simulink model "RedCrane_kinematic_model_telescope"  (R2024a)
settings: Solver=FixedStepAuto  StartTime=0.0  StopTime=40  FixedStep=Ts  MaxStep=0.005  RelTol=1e-3
values from neighbouring files (symbols this model uses):
  Cartesian_home = [3.55, 0.4, 1.6]'    [enviroment_setup.m]
  telescope0 = 0    [enviroment_setup.m]
  thetaList0 = [0, 0,-pi/8, 0, 0]'    [enviroment_setup.m]
  Ts = 0.001    [enviroment_setup.m]
undefined symbols (not defined in the file or in its folder): dp_k_angle_to_stroke, dp_m_angle_to_stroke, p_k_angle_to_stroke, p_k_stroke_to_angle, p_m_angle_to_stroke, p_m_stroke_to_angle, X, Y, Z
libraries: sm_lib x82, nesl_utility x19, fl_lib x16
(part 3 of 3)

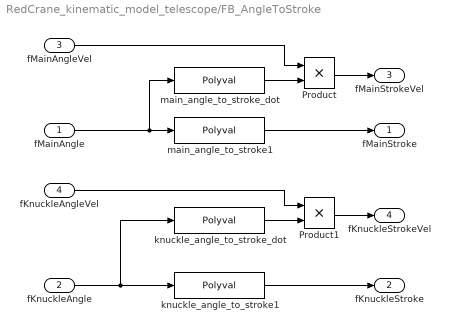
== system RedCrane_kinematic_model_telescope/FB_AngleToStroke ==
  fMainAngle : Inport
  fKnuckleAngle : Inport  Port=2
  fMainAngleVel : Inport  Port=3
  fKnuckleAngleVel : Inport  Port=4
  Product : Product
  Product1 : Product
  knuckle_angle_to_stroke1 : Polyval  Coefs=p_k_angle_to_stroke
  knuckle_angle_to_stroke_dot : Polyval  Coefs=dp_k_angle_to_stroke
  main_angle_to_stroke1 : Polyval  Coefs=p_m_angle_to_stroke
  main_angle_to_stroke_dot : Polyval  Coefs=dp_m_angle_to_stroke
  fMainStroke : Outport
  fKnuckleStroke : Outport  Port=2
  fMainStrokeVel : Outport  Port=3
  fKnuckleStrokeVel : Outport  Port=4
  wires:
  fMainAngle/1 -> main_angle_to_stroke_dot/1, main_angle_to_stroke1/1
  knuckle_angle_to_stroke_dot/1 -> Product1/2
  fKnuckleAngleVel/1 -> Product1/1
  fKnuckleAngle/1 -> knuckle_angle_to_stroke_dot/1, knuckle_angle_to_stroke1/1
  knuckle_angle_to_stroke1/1 -> fKnuckleStroke/1
  main_angle_to_stroke_dot/1 -> Product/2
  main_angle_to_stroke1/1 -> fMainStroke/1
  Product1/1 -> fKnuckleStrokeVel/1
  Product/1 -> fMainStrokeVel/1
  fMainAngleVel/1 -> Product/1

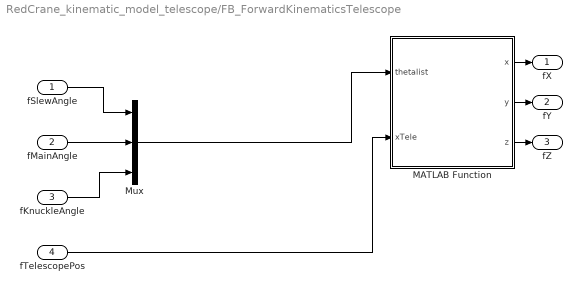
== system RedCrane_kinematic_model_telescope/FB_ForwardKinematicsTelescope ==
  fSlewAngle : Inport
  fMainAngle : Inport  Port=2
  fKnuckleAngle : Inport  Port=3
  fTelescopePos : Inport  Port=4
  MATLAB Function : MATLAB Function  TreatAsAtomicUnit=on
  Mux : Mux  Inputs=3
  fX : Outport
  fY : Outport  Port=2
  fZ : Outport  Port=3
  wires:
  MATLAB Function/1(x) -> fX/1
  fTelescopePos/1 -> MATLAB Function/2(xTele)
  Mux/1 -> MATLAB Function/1(thetalist)
  MATLAB Function/3(z) -> fZ/1
  MATLAB Function/2(y) -> fY/1
  fSlewAngle/1 -> Mux/1
  fMainAngle/1 -> Mux/2
  fKnuckleAngle/1 -> Mux/3

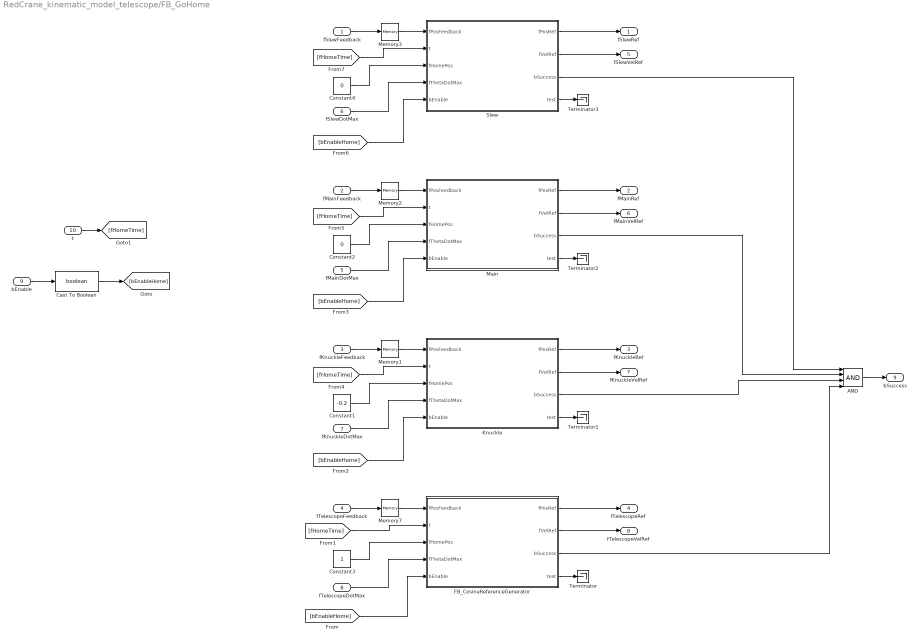
== system RedCrane_kinematic_model_telescope/FB_GoHome ==
  fSlewFeedback : Inport
  fMainFeedback : Inport  Port=2
  fKnuckleFeedback : Inport  Port=3
  fTelescopeFeedback : Inport  Port=4
  fMainDotMax : Inport  Port=5
  fSlewDotMax : Inport  Port=6
  fKnuckleDotMax : Inport  Port=7
  fTelescopeDotMax : Inport  Port=8
  bEnable : Inport  Port=9
  t : Inport  Port=10
  AND : Logic  Inputs=4  IconShape=distinctive  AllPortsSameDT=off  OutDataTypeStr=boolean
  Cast To Boolean : DataTypeConversion  OutDataTypeStr=boolean  SaturateOnIntegerOverflow=off  RndMeth=Floor
  Constant1 : Constant  Value=-0.2
  Constant2 : Constant  Value=0
  Constant3 : Constant
  Constant4 : Constant  Value=0
  FB_CosineReferenceGenerator : MATLAB Function  TreatAsAtomicUnit=on
  Knuckle : MATLAB Function  TreatAsAtomicUnit=on
  Main : MATLAB Function  TreatAsAtomicUnit=on
  Memory1 : Memory  InitialCondition=thetaList0(3)
  Memory2 : Memory  InitialCondition=thetaList0(2)
  Memory3 : Memory  InitialCondition=thetaList0(1)
  Memory7 : Memory  InitialCondition=telescope0
  Slew : MATLAB Function  TreatAsAtomicUnit=on
  Terminator{,1..3} (4 alike) : Terminator
  fSlewRef : Outport
  fMainRef : Outport  Port=2
  fKnuckleRef : Outport  Port=3
  fTelescopeRef : Outport  Port=4
  fSlewVelRef : Outport  Port=5
  fMainVelRef : Outport  Port=6
  fKnuckleVelRef : Outport  Port=7
  fTelescopeVelRef : Outport  Port=8
  bSuccess : Outport  Port=9
  wires:
  FB_CosineReferenceGenerator/1(fPosRef) -> fTelescopeRef/1
  FB_CosineReferenceGenerator/3(bSuccess) -> AND/4
  [fHomeTime] -> FB_CosineReferenceGenerator/2(t)
  fTelescopeDotMax/1 -> FB_CosineReferenceGenerator/4(fThetaDotMax)
  [bEnableHome] -> FB_CosineReferenceGenerator/5(bEnable)
  fTelescopeFeedback/1 -> Memory7/1
  Constant3/1 -> FB_CosineReferenceGenerator/3(fHomePos)
  Memory7/1 -> FB_CosineReferenceGenerator/1(fPosFeedback)
  FB_CosineReferenceGenerator/2(fVelRef) -> fTelescopeVelRef/1
  FB_CosineReferenceGenerator/4(test) -> Terminator/1
  Constant1/1 -> Knuckle/3(fHomePos)
  Knuckle/3(bSuccess) -> AND/3
  Knuckle/2(fVelRef) -> fKnuckleVelRef/1
  Memory1/1 -> Knuckle/1(fPosFeedback)
  Knuckle/4(test) -> Terminator1/1
  Knuckle/1(fPosRef) -> fKnuckleRef/1
  [bEnableHome] -> Knuckle/5(bEnable)
  fKnuckleDotMax/1 -> Knuckle/4(fThetaDotMax)
  [fHomeTime] -> Knuckle/2(t)
  fKnuckleFeedback/1 -> Memory1/1
  AND/1 -> bSuccess/1
  bEnable/1 -> Cast To Boolean/1
  t/1 -> [fHomeTime]
  Cast To Boolean/1 -> [bEnableHome]
  Main/3(bSuccess) -> AND/2
  fMainDotMax/1 -> Main/4(fThetaDotMax)
  Main/4(test) -> Terminator2/1
  fMainFeedback/1 -> Memory2/1
  Memory2/1 -> Main/1(fPosFeedback)
  Main/2(fVelRef) -> fMainVelRef/1
  [bEnableHome] -> Main/5(bEnable)
  Constant2/1 -> Main/3(fHomePos)
  Main/1(fPosRef) -> fMainRef/1
  [fHomeTime] -> Main/2(t)
  [bEnableHome] -> Slew/5(bEnable)
  Slew/2(fVelRef) -> fSlewVelRef/1
  Memory3/1 -> Slew/1(fPosFeedback)
  Slew/3(bSuccess) -> AND/1
  Slew/4(test) -> Terminator3/1
  [fHomeTime] -> Slew/2(t)
  Slew/1(fPosRef) -> fSlewRef/1
  fSlewFeedback/1 -> Memory3/1
  Constant4/1 -> Slew/3(fHomePos)
  fSlewDotMax/1 -> Slew/4(fThetaDotMax)

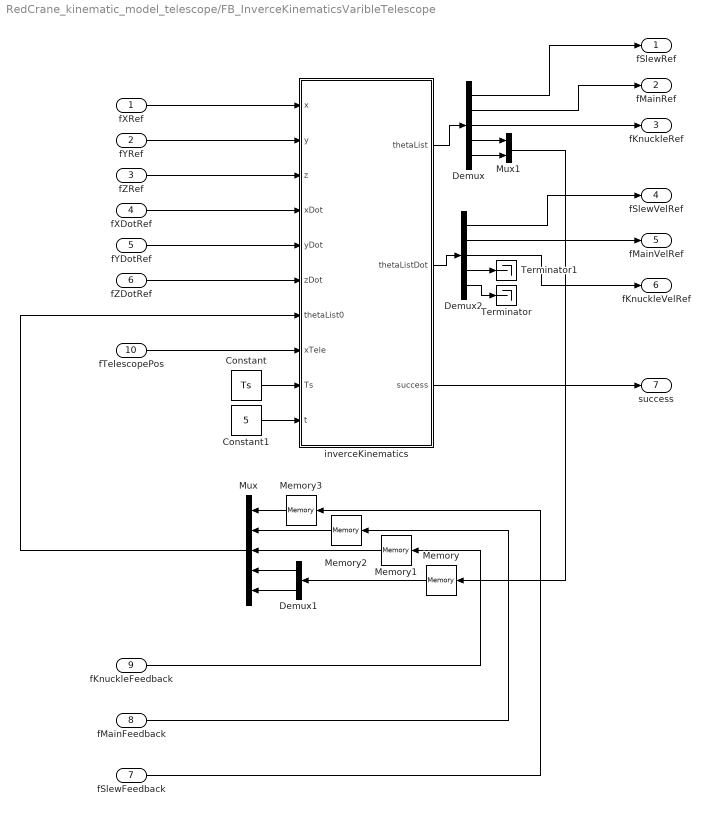
== system RedCrane_kinematic_model_telescope/FB_InverceKinematicsVaribleTelescope ==
  fXRef : Inport
  fYRef : Inport  Port=2
  fZRef : Inport  Port=3
  fXDotRef : Inport  Port=4
  fYDotRef : Inport  Port=5
  fZDotRef : Inport  Port=6
  fSlewFeedback : Inport  Port=7
  fMainFeedback : Inport  Port=8
  fKnuckleFeedback : Inport  Port=9
  fTelescopePos : Inport  Port=10
  Constant : Constant  Value=Ts
  Constant1 : Constant  Value=5
  Demux : Demux  Outputs=5
  Demux1 : Demux  Outputs=2
  Demux2 : Demux  Outputs=5
  Memory : Memory  InitialCondition=[thetaList0(4), thetaList0(5)]'
  Memory1 : Memory  InitialCondition=thetaList0(3)
  Memory2 : Memory  InitialCondition=thetaList0(2)
  Memory3 : Memory  InitialCondition=thetaList0(1)
  Mux : Mux  Inputs=5
  Mux1 : Mux  Inputs=2
  Terminator : Terminator
  Terminator1 : Terminator
  inverceKinematics : MATLAB Function  TreatAsAtomicUnit=on
  fSlewRef : Outport
  fMainRef : Outport  Port=2
  fKnuckleRef : Outport  Port=3
  fSlewVelRef : Outport  Port=4
  fMainVelRef : Outport  Port=5
  fKnuckleVelRef : Outport  Port=6
  success : Outport  Port=7
  wires:
  Memory1/1 -> Mux/3
  Demux/5 -> Mux1/2
  Memory3/1 -> Mux/1
  Demux2/5 -> Terminator/1
  fSlewFeedback/1 -> Memory3/1
  Demux1/2 -> Mux/5
  Memory2/1 -> Mux/2
  Demux2/1 -> fSlewVelRef/1
  fXDotRef/1 -> inverceKinematics/4(xDot)
  inverceKinematics/1(thetaList) -> Demux/1
  Constant1/1 -> inverceKinematics/10(t)
  Demux/1 -> fSlewRef/1
  fXRef/1 -> inverceKinematics/1(x)
  Constant/1 -> inverceKinematics/9(Ts)
  Demux1/1 -> Mux/4
  Mux/1 -> inverceKinematics/7(thetaList0)
  Mux1/1 -> Memory/1
  fZRef/1 -> inverceKinematics/3(z)
  Memory/1 -> Demux1/1
  inverceKinematics/2(thetaListDot) -> Demux2/1
  Demux/4 -> Mux1/1
  Demux2/4 -> Terminator1/1
  fMainFeedback/1 -> Memory2/1
  fYRef/1 -> inverceKinematics/2(y)
  fKnuckleFeedback/1 -> Memory1/1
  Demux/3 -> fKnuckleRef/1
  fYDotRef/1 -> inverceKinematics/5(yDot)
  fZDotRef/1 -> inverceKinematics/6(zDot)
  Demux2/3 -> fKnuckleVelRef/1
  Demux/2 -> fMainRef/1
  Demux2/2 -> fMainVelRef/1
  inverceKinematics/3(success) -> success/1
  fTelescopePos/1 -> inverceKinematics/8(xTele)

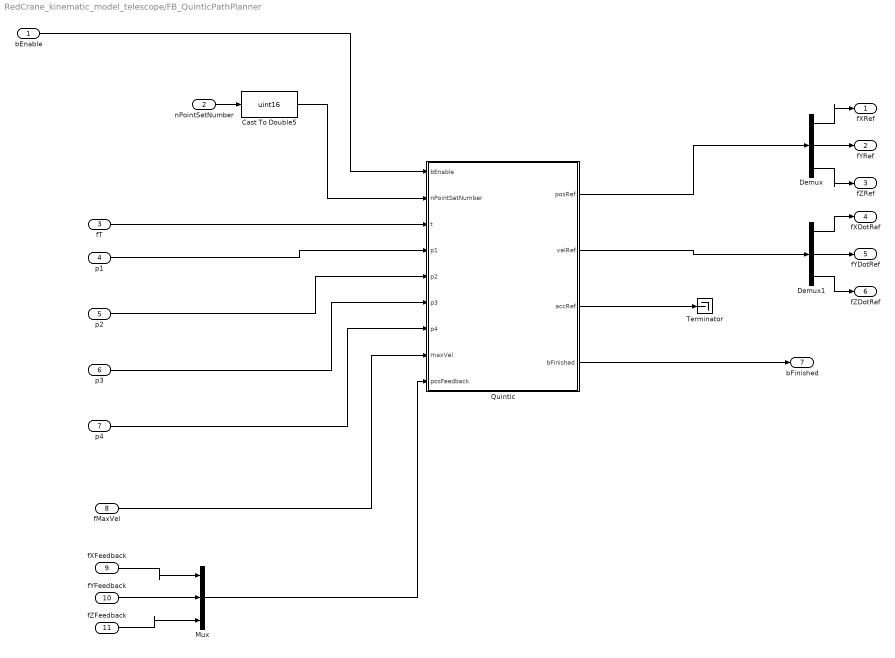
== system RedCrane_kinematic_model_telescope/FB_QuinticPathPlanner ==
  bEnable : Inport
  nPointSetNumber : Inport  Port=2
  fT : Inport  Port=3
  p1 : Inport  Port=4
  p2 : Inport  Port=5
  p3 : Inport  Port=6
  p4 : Inport  Port=7
  fMaxVel : Inport  Port=8
  fXFeedback : Inport  Port=9
  fYFeedback : Inport  Port=10
  fZFeedback : Inport  Port=11
  Cast To Double5 : DataTypeConversion  OutDataTypeStr=uint16  SaturateOnIntegerOverflow=off  RndMeth=Floor
  Demux : Demux  Outputs=3
  Demux1 : Demux  Outputs=3
  Mux : Mux  Inputs=3
  Quintic : MATLAB Function  TreatAsAtomicUnit=on
  Terminator : Terminator
  fXRef : Outport
  fYRef : Outport  Port=2
  fZRef : Outport  Port=3
  fXDotRef : Outport  Port=4
  fYDotRef : Outport  Port=5
  fZDotRef : Outport  Port=6
  bFinished : Outport  Port=7
  wires:
  fT/1 -> Quintic/3(t)
  p2/1 -> Quintic/5(p2)
  bEnable/1 -> Quintic/1(bEnable)
  fMaxVel/1 -> Quintic/8(maxVel)
  Quintic/4(bFinished) -> bFinished/1
  Quintic/1(posRef) -> Demux/1
  Quintic/3(accRef) -> Terminator/1
  p1/1 -> Quintic/4(p1)
  p3/1 -> Quintic/6(p3)
  p4/1 -> Quintic/7(p4)
  Mux/1 -> Quintic/9(posFeedback)
  nPointSetNumber/1 -> Cast To Double5/1
  Cast To Double5/1 -> Quintic/2(nPointSetNumber)
  Demux/2 -> fYRef/1
  Demux/1 -> fXRef/1
  Demux/3 -> fZRef/1
  Demux1/1 -> fXDotRef/1
  Demux1/2 -> fYDotRef/1
  Demux1/3 -> fZDotRef/1
  Quintic/2(velRef) -> Demux1/1
  fXFeedback/1 -> Mux/1
  fYFeedback/1 -> Mux/2
  fZFeedback/1 -> Mux/3

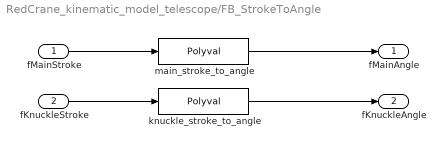
== system RedCrane_kinematic_model_telescope/FB_StrokeToAngle ==
  fMainStroke : Inport
  fKnuckleStroke : Inport  Port=2
  knuckle_stroke_to_angle : Polyval  Coefs=p_k_stroke_to_angle
  main_stroke_to_angle : Polyval  Coefs=p_m_stroke_to_angle
  fMainAngle : Outport
  fKnuckleAngle : Outport  Port=2
  wires:
  fKnuckleStroke/1 -> knuckle_stroke_to_angle/1
  fMainStroke/1 -> main_stroke_to_angle/1
  main_stroke_to_angle/1 -> fMainAngle/1
  knuckle_stroke_to_angle/1 -> fKnuckleAngle/1

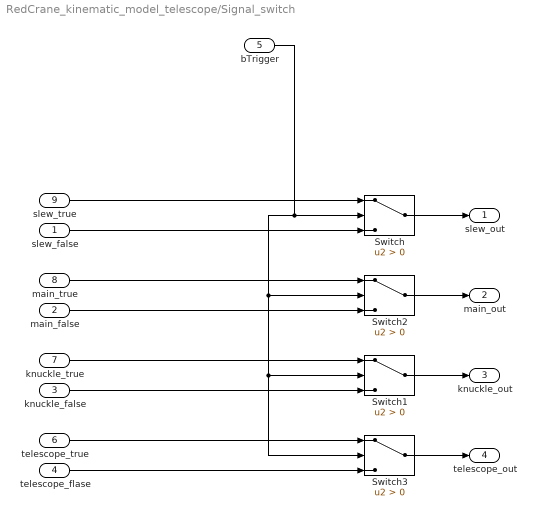
== system RedCrane_kinematic_model_telescope/Signal_switch ==
  slew_false : Inport
  main_false : Inport  Port=2
  knuckle_false : Inport  Port=3
  telescope_flase : Inport  Port=4
  bTrigger : Inport  Port=5
  telescope_true : Inport  Port=6
  knuckle_true : Inport  Port=7
  main_true : Inport  Port=8
  slew_true : Inport  Port=9
  Switch{,1..3} (4 alike) : Switch  Criteria=u2 > Threshold  SaturateOnIntegerOverflow=off  InputSameDT=off
  slew_out : Outport
  main_out : Outport  Port=2
  knuckle_out : Outport  Port=3
  telescope_out : Outport  Port=4
  wires:
  Switch1/1 -> knuckle_out/1
  bTrigger/1 -> Switch2/2, Switch1/2, Switch3/2, Switch/2
  telescope_true/1 -> Switch3/1
  slew_false/1 -> Switch/3
  Switch2/1 -> main_out/1
  slew_true/1 -> Switch/1
  knuckle_true/1 -> Switch1/1
  Switch3/1 -> telescope_out/1
  main_false/1 -> Switch2/3
  Switch/1 -> slew_out/1
  telescope_flase/1 -> Switch3/3
  knuckle_false/1 -> Switch1/3
  main_true/1 -> Switch2/1

== matlab function RedCrane_kinematic_model_telescope/FB_ForwardKinematicsTelescope/MATLAB Function ==
  data: thetalist input; x output; xTele input; y output; z output
function [x, y, z] = forvardKinematics(thetalist, xTele)

%% Deffine zero configuration trasform and screw axis with telescope
% Lengths
L1 = 250/1000; 
L2 = 1568.50/1000; 
L3 = 69.97/1000;
L4 = 2400/1000; 
L5 = 2428.99/1000; 
L6 = 92.52/1000;
L7 = 336.2/1000;

% Adjusting L5 based on telescope extention:
L5 = L5 + xTele;

% zero configuration trasform
M = [1, 0, 0, (L5 + L4 - L1);
    0, 1, 0 (L7);
    0, 0, 1, (L2+ L3 - L6);
    0, 0, 0, 1];

% screw axis
ws1 = [0, 0, 1]';
ws2 = [0, -1, 0]';
ws3 = [0, -1, 0]';
ws4 = [0, 1, 0]';
ws5 = [0, 0, 1]';

% coordinates of an arbitrary point along the screw axis
qs1 = [0, 0, 0]';
qs2 = [-L1, 0, L2]';
qs3 = [(L4 - L1), 0, (L2 + L3)]';
qs4 = [(L5 + L4 - L1), L7, (L2 + L3 - L6)]';
qs5 = qs4;

% Building screw axis matrix
ws_mat = [ws1, ws2, ws3, ws4, ws5];
vs_mat = [cross(qs1, ws1), cross(qs2, ws2), ...
          cross(qs3, ws3), cross(qs4, ws4), ...
          cross(qs5, ws5)];

SList = [ws_mat;
    vs_mat];

T = zeros(4, 4);
T = FKinSpace(M, SList, thetalist);

x = T(1, 4);
y = T(2, 4);
z = T(3, 4);

== matlab function RedCrane_kinematic_model_telescope/FB_QuinticPathPlanner/Quintic ==
  settings: updateMethod=DISCRETE
  data: bEnable input; nPointSetNumber input; posRef output; t input; velRef output; accRef output; p1 input; p2 input; p3 input; p4 input; maxVel input; bFinished output; posFeedback input
function [posRef, velRef, accRef, bFinished] = QuinticGenerator( ...
    bEnable, nPointSetNumber, t, p1, p2, p3, p4, maxVel, posFeedback )
% QUINTICGENERATOR
%   Generates piecewise polynomial references (pos/vel/acc) for up to 4 segments.
%   Re-computes polynomials only when nPointSetNumber increments (signaling
%   a new waypoint set), and only if bEnable == true.
%
%   If bEnable is false, outputs a stationary reference at posFeedback.

    %%% PERSISTENT VARIABLES %%%%%%%%%%%%%%%%%%%%%%%%%%%%%%%%%%%%%%%%%%%%%
    persistent bEnableMemory                % Remember last enable state
    persistent pointSetNumberMemory         % Remember last waypoint-set counter
    
    persistent p1Memory p2Memory p3Memory p4Memory
    persistent timeSlotsMemory
    persistent coeffXMemory coeffYMemory coeffZMemory
    persistent posRefMemory velRefMemory accRefMemory
    persistent t0Memory                    % Local start time offset
    
    % Initialize persistent variables if empty
    if isempty(bEnableMemory),       bEnableMemory       = false;      end
    if isempty(pointSetNumberMemory),pointSetNumberMemory= uint16(0);  end
    
    if isempty(p1Memory),           p1Memory            = zeros(3,1); end
    if isempty(p2Memory),           p2Memory            = zeros(3,1); end
    if isempty(p3Memory),           p3Memory            = zeros(3,1); end
    if isempty(p4Memory),           p4Memory            = zeros(3,1); end
    
    if isempty(timeSlotsMemory),     timeSlotsMemory     = [0 1 2 3 4];end
    if isempty(coeffXMemory),        coeffXMemory        = zeros(18,1);end
    if isempty(coeffYMemory),        coeffYMemory        = zeros(18,1);end
    if isempty(coeffZMemory),        coeffZMemory        = zeros(18,1);end
    
    if isempty(posRefMemory),        posRefMemory        = posFeedback; end
    if isempty(velRefMemory),        velRefMemory        = zeros(3,1); end
    if isempty(accRefMemory),        accRefMemory        = zeros(3,1); end
    
    if isempty(t0Memory),           t0Memory            = 0;          end

    %%% DEFAULT OUTPUTS (if bEnable == false) %%%%%%%%%%%%%%%%%%%%%%%%%%%%
    %   Stationary reference at the current feedback position
    posRef    = posFeedback;   
    velRef    = zeros(3,1);
    accRef    = zeros(3,1);
    bFinished = true;  % Not actively running any trajectory
    bFirsCykle = false;
    %----------------------------------------------------------------------
    % 1) CHECK IF DISABLED => Return a stationary reference immediately
    %----------------------------------------------------------------------
    if ~bEnable
        % Make sure to remember we are now disabled
        bEnableMemory = false;
        return;
    end

    %----------------------------------------------------------------------
    % 2) IF WE GET HERE => bEnable == true
    %    We want to see if we just transitioned from false->true
    %----------------------------------------------------------------------
    if bEnable && ~bEnableMemory
        % Rising edge of bEnable => reset local start time
        %t0Memory = t;
        bFirsCykle = true;
    end
    
    % Update bEnableMemory to reflect the current state
    bEnableMemory = true;

    %----------------------------------------------------------------------
    % 3) Check if nPointSetNumber has incremented => new waypoints
    %----------------------------------------------------------------------
    if nPointSetNumber > pointSetNumberMemory
        bNewPointSet = true;
        pointSetNumberMemory = nPointSetNumber;
    else
        bNewPointSet = false;
    end
        
    %reset local start time
    if bFirsCykle | bNewPointSet
        t0Memory = t;
    end


    %----------------------------------------------------------------------
    % 4) If new points, compute new polynomials
    %    We only do this if we are enabled (which we are) 
    %----------------------------------------------------------------------
    if bNewPointSet
        % Save new waypoints
        p1Memory = p1;
        p2Memory = p2;
        p3Memory = p3;
        p4Memory = p4;
        
        % We can choose velocity/accel for start from the *old* memory 
        % or from zero. Example: from memory
        v0x = velRefMemory(1);  a0x = accRefMemory(1);
        v0y = velRefMemory(2);  a0y = accRefMemory(2);
        v0z = velRefMemory(3);  a0z = accRefMemory(3);

        % Build vectors of 5 points in each dimension
        % Start from the current feedback (or last posRefMemory),
        % but commonly we use posFeedback for a fresh start.
        xPoints = [posFeedback(1), p1(1), p2(1), p3(1), p4(1)];
        yPoints = [posFeedback(2), p1(2), p2(2), p3(2), p4(2)];
        zPoints = [posFeedback(3), p1(3), p2(3), p3(3), p4(3)];

        % Time computations
        maxVel3D = maxVel / sqrt(3);  % if you want sqrt(vx^2 + vy^2 + vz^2) = maxVel
        dTemp1 = [xPoints(1), yPoints(1), zPoints(1)] - [xPoints(2), yPoints(2), zPoints(2)];
        dTemp2 = [xPoints(2), yPoints(2), zPoints(2)] - [xPoints(3), yPoints(3), zPoints(3)];
        dTemp3 = [xPoints(3), yPoints(3), zPoints(3)] - [xPoints(4), yPoints(4), zPoints(4)];
        dTemp4 = [xPoints(4), yPoints(4), zPoints(4)] - [xPoints(5), yPoints(5), zPoints(5)];

        t1 = norm(dTemp1) / maxVel3D;
        t2 = norm(dTemp2) / maxVel3D;
        t3 = norm(dTemp3) / maxVel3D;
        t4 = norm(dTemp4) / maxVel3D;
        
        timeSlots = [0, t1, t1 + t2, t1 + t2 + t3, t1 + t2 + t3 + t4];
        timeSlotsMemory = timeSlots;

        % Compute polynomials (Quintic)
        coeffX = Quintic(timeSlots, xPoints, v0x, a0x);
        coeffY = Quintic(timeSlots, yPoints, v0y, a0y);
        coeffZ = Quintic(timeSlots, zPoints, v0z, a0z);
        
        coeffXMemory = coeffX;
        coeffYMemory = coeffY;
        coeffZMemory = coeffZ;
    end

    %----------------------------------------------------------------------
    % 5) Evaluate polynomials at local time => tLocal = t - t0Memory
    %----------------------------------------------------------------------
    tLocal = t - t0Memory;

    % If local time is beyond the final timeSlot => clamp & declare finished
    timeSlots = timeSlotsMemory;
    if tLocal >= timeSlots(end)
        tLocal = timeSlots(end);
        bFinished = true;
    else
        bFinished = false;
    end

    % Retrieve precomputed coefficients
    coeffX = coeffXMemory;
    coeffY = coeffYMemory;
    coeffZ = coeffZMemory;

    % Decide which segment to evaluate
    if tLocal < timeSlots(2)
        % Segment 1 (4th order)
        posRef = [F4(tLocal)*coeffX(1:5);
                  F4(tLocal)*coeffY(1:5);
                  F4(tLocal)*coeffZ(1:5)];

        velRef = [F4Dot(tLocal)*coeffX(1:5);
                  F4Dot(tLocal)*coeffY(1:5);
                  F4Dot(tLocal)*coeffZ(1:5)];

        accRef = [F4DotDot(tLocal)*coeffX(1:5);
                  F4DotDot(tLocal)*coeffY(1:5);
                  F4DotDot(tLocal)*coeffZ(1:5)];

    elseif tLocal < timeSlots(3)
        % Segment 2 (3rd order)
        posRef = [F3(tLocal)*coeffX(6:9);
                  F3(tLocal)*coeffY(6:9);
                  F3(tLocal)*coeffZ(6:9)];

        velRef = [F3Dot(tLocal)*coeffX(6:9);
                  F3Dot(tLocal)*coeffY(6:9);
                  F3Dot(tLocal)*coeffZ(6:9)];

        accRef = [F3DotDot(tLocal)*coeffX(6:9);
                  F3DotDot(tLocal)*coeffY(6:9);
                  F3DotDot(tLocal)*coeffZ(6:9)];

    elseif tLocal < timeSlots(4)
        % Segment 3 (3rd order)
        posRef = [F3(tLocal)*coeffX(10:13);
                  F3(tLocal)*coeffY(10:13);
                  F3(tLocal)*coeffZ(10:13)];

        velRef = [F3Dot(tLocal)*coeffX(10:13);
                  F3Dot(tLocal)*coeffY(10:13);
                  F3Dot(tLocal)*coeffZ(10:13)];

        accRef = [F3DotDot(tLocal)*coeffX(10:13);
                  F3DotDot(tLocal)*coeffY(10:13);
                  F3DotDot(tLocal)*coeffZ(10:13)];
              
    else
        % Segment 4 (4th order)
        posRef = [F4(tLocal)*coeffX(14:18);
                  F4(tLocal)*coeffY(14:18);
                  F4(tLocal)*coeffZ(14:18)];

        velRef = [F4Dot(tLocal)*coeffX(14:18);
                  F4Dot(tLocal)*coeffY(14:18);
                  F4Dot(tLocal)*coeffZ(14:18)];

        accRef = [F4DotDot(tLocal)*coeffX(14:18);
                  F4DotDot(tLocal)*coeffY(14:18);
                  F4DotDot(tLocal)*coeffZ(14:18)];
    end

    %----------------------------------------------------------------------
    % 6) Save references to memory for next cycle
    %----------------------------------------------------------------------
    posRefMemory = posRef;
    velRefMemory = velRef;
    accRefMemory = accRef;

end

== matlab function RedCrane_kinematic_model_telescope/FB_GoHome/Knuckle ==
  settings: updateMethod=DISCRETE
  data: fPosRef output; fVelRef output; fPosFeedback input; t input; fHomePos input; bSuccess output; fThetaDotMax input; bEnable input; test output
function [fPosRef, fVelRef, bSuccess, test] = goHomeKnuckle(fPosFeedback, ...
    t,...
    fHomePos,...
    fThetaDotMax, ...
    bEnable)

bSuccess = false;
fPosRef = 0.0;
fVelRef = 0.0;
test = false;




[fPosRef, fVelRef, bSuccess, test] = cosinePositionGenerator(fPosFeedback, fHomePos, fThetaDotMax, t, bEnable);



end

== matlab function RedCrane_kinematic_model_telescope/FB_InverceKinematicsVaribleTelescope/inverceKinematics ==
  data: x input; thetaList output size=[5, 1]; y input; z input; xDot input; yDot input; zDot input; thetaList0 input; xTele input; Ts input; thetaListDot output size=[5, 1]; success output size=1; t input
function [thetaList, thetaListDot, success] = inverceKinematics( ...
    x, y, z, xDot, yDot, zDot, thetaList0, xTele, Ts, t)

if(t <= Ts*1.1)
    thetaList0 = [0, 0, 0, 0, 0]';
end

%% Deffine zero configuration trasform and screw axis with telescope
% Lengths
L1 = 250/1000; 
L2 = 1568.50/1000; 
L3 = 69.97/1000;
L4 = 2400/1000; 
L5 = 2428.99/1000; 
L6 = 92.52/1000;
L7 = 336.2/1000;

% Adjusting L5 based on telescope extention:
L5 = L5 + xTele;

% zero configuration trasform
M = [1, 0, 0, (L5 + L4 - L1);
    0, 1, 0 (L7);
    0, 0, 1, (L2+ L3 - L6);
    0, 0, 0, 1];

% screw axis
ws1 = [0, 0, 1]';
ws2 = [0, -1, 0]';
ws3 = [0, -1, 0]';
ws4 = [0, 1, 0]';
ws5 = [0, 0, 1]';

% coordinates of an arbitrary point along the screw axis
qs1 = [0, 0, 0]';
qs2 = [-L1, 0, L2]';
qs3 = [(L4 - L1), 0, (L2 + L3)]';
qs4 = [(L5 + L4 - L1), L7, (L2 + L3 - L6)]';
qs5 = qs4;

% Building screw axis matrix
ws_mat = [ws1, ws2, ws3, ws4, ws5];
vs_mat = [cross(qs1, ws1), cross(qs2, ws2), ...
          cross(qs3, ws3), cross(qs4, ws4), ...
          cross(qs5, ws5)];

SList = [ws_mat;
    vs_mat];


%%
% Explicitly pre-assign outputs
thetaList    = zeros(5,1);
thetaListDot = zeros(5,1);
success      = false;    % or 0 if you prefer numeric


T = [1 0 0 x;
    0 1 0 y;
    0 0 1 z;
    0 0 0 1];


[thetaOut, successOut] = IKinSpace(SList, M, T, thetaList0, 0.00001, 0.0000001);

% Assign them to the pre-allocated outputs
thetaList    = thetaOut;
success      = successOut;


Js = JacobianSpace(SList,thetaList);
Js_pinv = pinv(Js);
xyzDot = [0;
         0;
         0;
         xDot;
         yDot;
         zDot
         ];

thetaListDot = Js_pinv*xyzDot;

end

== matlab function RedCrane_kinematic_model_telescope/FB_GoHome/Main ==
  settings: updateMethod=DISCRETE
  data: fPosRef output; fVelRef output; fPosFeedback input; t input; fHomePos input; bSuccess output; fThetaDotMax input; bEnable input; test output
function [fPosRef, fVelRef, bSuccess, test] = goHomeMain(fPosFeedback, ...
    t,...
    fHomePos,...
    fThetaDotMax, ...
    bEnable)

bSuccess = false;
fPosRef = 0.0;
fVelRef = 0.0;
test = false;




[fPosRef, fVelRef, bSuccess, test] = cosinePositionGenerator(fPosFeedback, fHomePos, fThetaDotMax, t, bEnable);



end

== matlab function RedCrane_kinematic_model_telescope/FB_GoHome/Slew ==
  settings: updateMethod=DISCRETE
  data: fPosRef output; fVelRef output; fPosFeedback input; t input; fHomePos input; bSuccess output; fThetaDotMax input; bEnable input; test output
function [fPosRef, fVelRef, bSuccess, test] = goHomeSlew(fPosFeedback, ...
    t,...
    fHomePos,...
    fThetaDotMax, ...
    bEnable)

bSuccess = false;
fPosRef = 0.0;
fVelRef = 0.0;
test = false;




[fPosRef, fVelRef, bSuccess, test] = cosinePositionGenerator(fPosFeedback, fHomePos, fThetaDotMax, t, bEnable);



end

== matlab function RedCrane_kinematic_model_telescope/FB_GoHome/FB_CosineReferenceGenerator ==
  settings: updateMethod=DISCRETE
  data: fPosRef output; fVelRef output; fPosFeedback input; t input; fHomePos input; bSuccess output; fThetaDotMax input; bEnable input; test output
function [fPosRef, fVelRef, bSuccess, test] = goHomeTelescope(fPosFeedback, ...
    t,...
    fHomePos,...
    fThetaDotMax, ...
    bEnable)

bSuccess = false;
fPosRef = 0.0;
fVelRef = 0.0;
test = false;


[fPosRef, fVelRef, bSuccess, test] = cosinePositionGenerator(fPosFeedback, fHomePos, fThetaDotMax, t, bEnable);



end

== matlab function RedCrane_kinematic_model_telescope/MATLAB Function ==
  data: xRef input; distance output; yRef input; zRef input; a output; xt output; L5 input; desiredKnuckleAngleDeg input
function [distance, a, xt]  = fcn(xRef, yRef, zRef, L5, desiredKnuckleAngleDeg)
%% Destacne between main joint and desirex (y, y, z)
roA = [0, 0, 1.5685]'; % Approximate vector from orego to main joint
roP = [xRef, yRef, zRef]'; % Vector from orego to desired point
distance = norm(roA - roP);
xt = 0;
%L5 = 2.3;
% Using law of cosine:
b = 2.4; % Length between main joint and knuckle joint
C = deg2rad(desiredKnuckleAngleDeg); % Desired knuckle angle
c = distance;

if ((c^2 -b^2 + b^2*(cos(C))^2)) <= 0.0
    a = 0;
    return
end
a = b*cos(C) + sqrt(c^2 -b^2 + b^2*(cos(C))^2);
xt = max(0, (a - L5));

end
